simulink model "dspwlet"  (Simulink 6.0)
settings: Solver=FixedStepDiscrete  StartTime=0.0  StopTime=2*length(lor)  RelTol=1e-3
PreLoadFcn:
  | load dspwlets;
values from neighbouring files (symbols this model uses):
  ts = [-1 0]    [lmsxy.m]    (also in sdspwwvdisp.m = get_param(blk,'CompiledSampleTime'))
undefined symbols (not defined in the file or in its folder): lor
libraries: dspmlti3 x6, dspsrcs4 x1
settings Model: Creator=don  LastModifiedBy=schim  ExtModeTrigMode=oneshot  ExtModeArmWhenConnect=off
settings DataIOCC: LimitDataPoints=off  SaveOutput=off  SaveTime=off  SignalLoggingName=logsOut
settings OptimizationCC: BooleanDataType=off  RollThreshold=2
settings DebuggingCC: CheckExecutionContextPreStartOutputMsg=on  CheckExecutionContextRuntimeOutputMsg=on  SolverPrmCheckMsg=none  IntegerOverflowMsg=none
settings HardwareCC: TargetUnknown=on
settings SFSimCC: SFSimApplyToAllLibs=on  SFSimBuildMode=Incremental

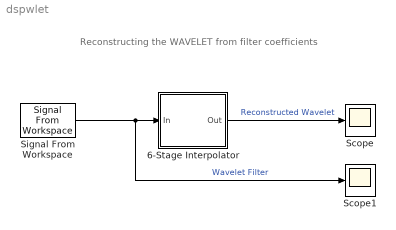
== system dspwlet ==
  note: Reconstructing the WAVELET
      | from filter coefficients
  6-Stage Interpolator : Subsystem  PropExecContextAcrossSSBoundary=on
  Scope : Scope
      settings: TimeRange=16  YMin=-0.0015  YMax=0.002  DataFormat=Array
  Scope1 : Scope
      settings: TimeRange=16  YMin=-0.8  YMax=0.8  DataFormat=Array
  Signal From Workspace : dspsrcs4/Signal From Workspace  X=hir  Ts=ts  nsamps=1  OutputAfterFinalValue=Setting to zero
  wires:
  Signal From Workspace/1 -> 6-Stage Interpolator/1(In), Scope1/1  "Wavelet Filter"
  6-Stage Interpolator/1(Out) -> Scope/1  "Reconstructed Wavelet"

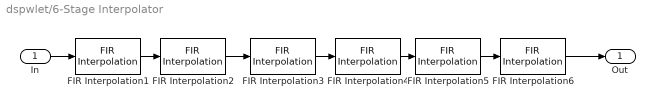
== system dspwlet/6-Stage Interpolator ==
  In : Inport  LatchInput=off
  FIR Interpolation1 : dspmlti3/FIR Interpolation  DialogController=dspDDGCreate  DialogControllerArgs=DataTag0  h=lor./2  L=2  framing=Maintain input frame size  outputBufInitCond=0  roundingMode=Floor  overflowMode=off
  FIR Interpolation2 : dspmlti3/FIR Interpolation  DialogController=dspDDGCreate  DialogControllerArgs=DataTag1  h=lor./2  L=2  framing=Maintain input frame size  outputBufInitCond=0  roundingMode=Floor  overflowMode=off
  FIR Interpolation3 : dspmlti3/FIR Interpolation  DialogController=dspDDGCreate  DialogControllerArgs=DataTag2  h=lor./2  L=2  framing=Maintain input frame size  outputBufInitCond=0  roundingMode=Floor  overflowMode=off
  FIR Interpolation4 : dspmlti3/FIR Interpolation  DialogController=dspDDGCreate  DialogControllerArgs=DataTag3  h=lor./2  L=2  framing=Maintain input frame size  outputBufInitCond=0  roundingMode=Floor  overflowMode=off
  FIR Interpolation5 : dspmlti3/FIR Interpolation  DialogController=dspDDGCreate  DialogControllerArgs=DataTag4  h=lor./2  L=2  framing=Maintain input frame size  outputBufInitCond=0  roundingMode=Floor  overflowMode=off
  FIR Interpolation6 : dspmlti3/FIR Interpolation  DialogController=dspDDGCreate  DialogControllerArgs=DataTag5  h=lor./2  L=2  framing=Maintain input frame size  outputBufInitCond=0  roundingMode=Floor  overflowMode=off
  Out : Outport
  wires:
  FIR Interpolation1/1 -> FIR Interpolation2/1
  FIR Interpolation2/1 -> FIR Interpolation3/1
  FIR Interpolation3/1 -> FIR Interpolation4/1
  FIR Interpolation4/1 -> FIR Interpolation5/1
  FIR Interpolation5/1 -> FIR Interpolation6/1
  FIR Interpolation6/1 -> Out/1
  In/1 -> FIR Interpolation1/1
